simulink model "PruebaSS"  (R2022a)
settings: Solver=VariableStepAuto  StartTime=0.0  StopTime=inf  RelTol=1e-3
values from neighbouring files (symbols this model uses):
  a = 0.2    [Data.m]
  alturaobst = 0.9    [Data.m]
  b = 0.542    [Data.m]
  Ki = 2.88815347475101    (= 2.88815347475)    [Data.m]
  Kp = 0.135293078315631    (= 0.135293078316)    [Data.m]
  M = [x_new y_new]    [Data.m]
  M_chasis = 3.5    [Data.m]
  M_rueda = 1    [Data.m]
  M_ruedacontacto = 1    [Data.m]
  N = 4365    [GraficasVelocidades.m]    (also in Prueba_Liapunov.m = length(p_X); WaypointsToTrayectory.m = length(X))
  posBordes = [xobstac, yobstac; xp1, yobstac; xp2, yobstac; xobstac, yp1; xobstac, yp2 ... (first row only)    [Data.m]
  pruebaM = WaypointsToTrayectory(prue,div)    [Data.m]
  R = 0.175/2    (= 0.0875)    [Data.m]
  X = M(:,1)    [WaypointsToTrayectory.m]
  x0 = x_ini(1)*factorE    [Data.m]
  x_obj = pos_fin(1)*factorE    [Data.m]
  xobstac = RandomPos(1)    [Data.m]
  Y = M(:, 2)    [WaypointsToTrayectory.m]
  y0 = y_ini(2)*factorE    [Data.m]
  y_obj = pos_fin(2)*factorE    [Data.m]
  yobstac = RandomPos(2)    [Data.m]
  zobstac = RandomPos(3)    [Data.m]
undefined symbols (not defined in the file or in its folder): bloqueobstaculo, Borde11, Borde12, Borde2, Borde3, Borde41, Borde42, Explanada, Kd, plano150g1, plano150g2, plano150g3, plano150g4, Plano150mm, plano150mm2irr, Plano45mm, plano45mm2irr, Plano90mm, Rampa, Rampa21, Rampa22, Rampa31, Rampa32, Rampa33, Rampa4, Rampa51, Rampa52, Rampa53, Terreno, Z
libraries: sm_lib x333, nesl_utility x29, fl_lib x3, slpidlib x2, robotalgslib x2
(part 7 of 7)

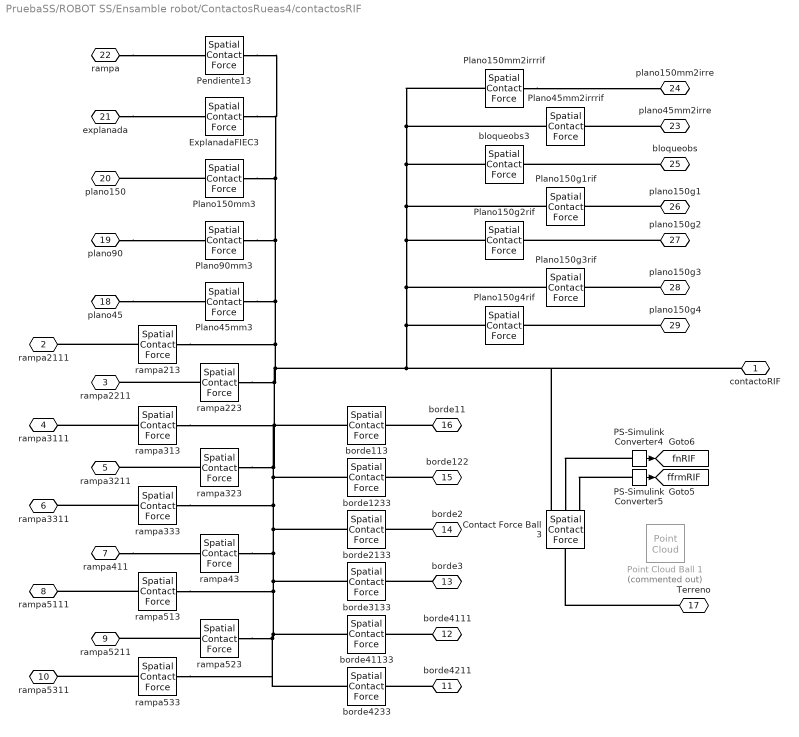
== system PruebaSS/ROBOT SS/Ensamble robot/ContactosRueas4/contactosRIF ==
  Contact Force Ball 3 : sm_lib/Forces and Torques/Spatial Contact Force  SenseContactBaseRotation=off  SenseContactBaseTranslation=off  CoefficientOfDynamicFriction=0.5  CoefficientOfStaticFriction=0.8  NormalDamping=1000  NormalDampingUnits=N/(m/s)  SenseContactSignal=off  NormalStiffness=1000000  NormalStiffnessUnits=N/m  FrictionalCriticalVelocity=1e-3  FrictionalCriticalVelocityUnits=m/s  ZeroCrossDetectContactStartAndEnd=off  SenseContactFollowerRotation=off  SenseContactFollowerTranslation=off  FrictionType=SmoothStickSlip  SenseFrictionalForceMagnitude=on  SenseNormalForceMagnitude=on  NormalForceType=SmoothSpringDamper  SenseNormalVelocity=off  SenseSeparationDistance=off  SenseTangentialVelocity=off  NormalTransitionRegionWidth=1e-4  NormalTransitionRegionWidthUnits=m
  ExplanadaFIEC3 : sm_lib/Forces and Torques/Spatial Contact Force  SenseContactBaseRotation=off  SenseContactBaseTranslation=off  CoefficientOfDynamicFriction=0.3  CoefficientOfStaticFriction=0.5  NormalDamping=1e3  NormalDampingUnits=N/(m/s)  SenseContactSignal=off  NormalStiffness=1e6  NormalStiffnessUnits=N/m  FrictionalCriticalVelocity=1e-3  FrictionalCriticalVelocityUnits=m/s  ZeroCrossDetectContactStartAndEnd=off  SenseContactFollowerRotation=off  SenseContactFollowerTranslation=off  FrictionType=SmoothStickSlip  SenseFrictionalForceMagnitude=off  SenseNormalForceMagnitude=off  NormalForceType=SmoothSpringDamper  SenseNormalVelocity=off  SenseSeparationDistance=off  SenseTangentialVelocity=off  NormalTransitionRegionWidth=1e-4  NormalTransitionRegionWidthUnits=m
  PS-Simulink Converter4 : nesl_utility/PS-Simulink Converter  PhysicalDomain=network_engine_domain  SubClassName=ps_output  LeftPortType=input  RightPortType=output  PseudoPeriodic=off  Frequencies=[]  VectorFormat=inherit  Unit=inherit  AffineConversion=off
      settings: SourceProductBaseCode=SS,PW,VE
  PS-Simulink Converter5 : nesl_utility/PS-Simulink Converter  PhysicalDomain=network_engine_domain  SubClassName=ps_output  LeftPortType=input  RightPortType=output  PseudoPeriodic=off  Frequencies=[]  VectorFormat=inherit  Unit=inherit  AffineConversion=off
      settings: SourceProductBaseCode=SS,PW,VE
  Pendiente13 : sm_lib/Forces and Torques/Spatial Contact Force  SenseContactBaseRotation=off  SenseContactBaseTranslation=off  CoefficientOfDynamicFriction=0.3  CoefficientOfStaticFriction=0.5  NormalDamping=1e3  NormalDampingUnits=N/(m/s)  SenseContactSignal=off  NormalStiffness=1e6  NormalStiffnessUnits=N/m  FrictionalCriticalVelocity=1e-3  FrictionalCriticalVelocityUnits=m/s  ZeroCrossDetectContactStartAndEnd=off  SenseContactFollowerRotation=off  SenseContactFollowerTranslation=off  FrictionType=SmoothStickSlip  SenseFrictionalForceMagnitude=off  SenseNormalForceMagnitude=off  NormalForceType=SmoothSpringDamper  SenseNormalVelocity=off  SenseSeparationDistance=off  SenseTangentialVelocity=off  NormalTransitionRegionWidth=1e-4  NormalTransitionRegionWidthUnits=m
  Plano150g1rif : sm_lib/Forces and Torques/Spatial Contact Force  SenseContactBaseRotation=off  SenseContactBaseTranslation=off  CoefficientOfDynamicFriction=0.3  CoefficientOfStaticFriction=0.5  NormalDamping=1e3  NormalDampingUnits=N/(m/s)  SenseContactSignal=off  NormalStiffness=1e6  NormalStiffnessUnits=N/m  FrictionalCriticalVelocity=1e-3  FrictionalCriticalVelocityUnits=m/s  ZeroCrossDetectContactStartAndEnd=off  SenseContactFollowerRotation=off  SenseContactFollowerTranslation=off  FrictionType=SmoothStickSlip  SenseFrictionalForceMagnitude=off  SenseNormalForceMagnitude=off  NormalForceType=SmoothSpringDamper  SenseNormalVelocity=off  SenseSeparationDistance=off  SenseTangentialVelocity=off  NormalTransitionRegionWidth=1e-4  NormalTransitionRegionWidthUnits=m
  Plano150g2rif : sm_lib/Forces and Torques/Spatial Contact Force  SenseContactBaseRotation=off  SenseContactBaseTranslation=off  CoefficientOfDynamicFriction=0.3  CoefficientOfStaticFriction=0.5  NormalDamping=1e3  NormalDampingUnits=N/(m/s)  SenseContactSignal=off  NormalStiffness=1e6  NormalStiffnessUnits=N/m  FrictionalCriticalVelocity=1e-3  FrictionalCriticalVelocityUnits=m/s  ZeroCrossDetectContactStartAndEnd=off  SenseContactFollowerRotation=off  SenseContactFollowerTranslation=off  FrictionType=SmoothStickSlip  SenseFrictionalForceMagnitude=off  SenseNormalForceMagnitude=off  NormalForceType=SmoothSpringDamper  SenseNormalVelocity=off  SenseSeparationDistance=off  SenseTangentialVelocity=off  NormalTransitionRegionWidth=1e-4  NormalTransitionRegionWidthUnits=m
  Plano150g3rif : sm_lib/Forces and Torques/Spatial Contact Force  SenseContactBaseRotation=off  SenseContactBaseTranslation=off  CoefficientOfDynamicFriction=0.3  CoefficientOfStaticFriction=0.5  NormalDamping=1e3  NormalDampingUnits=N/(m/s)  SenseContactSignal=off  NormalStiffness=1e6  NormalStiffnessUnits=N/m  FrictionalCriticalVelocity=1e-3  FrictionalCriticalVelocityUnits=m/s  ZeroCrossDetectContactStartAndEnd=off  SenseContactFollowerRotation=off  SenseContactFollowerTranslation=off  FrictionType=SmoothStickSlip  SenseFrictionalForceMagnitude=off  SenseNormalForceMagnitude=off  NormalForceType=SmoothSpringDamper  SenseNormalVelocity=off  SenseSeparationDistance=off  SenseTangentialVelocity=off  NormalTransitionRegionWidth=1e-4  NormalTransitionRegionWidthUnits=m
  Plano150g4rif : sm_lib/Forces and Torques/Spatial Contact Force  SenseContactBaseRotation=off  SenseContactBaseTranslation=off  CoefficientOfDynamicFriction=0.3  CoefficientOfStaticFriction=0.5  NormalDamping=1e3  NormalDampingUnits=N/(m/s)  SenseContactSignal=off  NormalStiffness=1e6  NormalStiffnessUnits=N/m  FrictionalCriticalVelocity=1e-3  FrictionalCriticalVelocityUnits=m/s  ZeroCrossDetectContactStartAndEnd=off  SenseContactFollowerRotation=off  SenseContactFollowerTranslation=off  FrictionType=SmoothStickSlip  SenseFrictionalForceMagnitude=off  SenseNormalForceMagnitude=off  NormalForceType=SmoothSpringDamper  SenseNormalVelocity=off  SenseSeparationDistance=off  SenseTangentialVelocity=off  NormalTransitionRegionWidth=1e-4  NormalTransitionRegionWidthUnits=m
  Plano150mm2irrrif : sm_lib/Forces and Torques/Spatial Contact Force  SenseContactBaseRotation=off  SenseContactBaseTranslation=off  CoefficientOfDynamicFriction=0.3  CoefficientOfStaticFriction=0.5  NormalDamping=1e3  NormalDampingUnits=N/(m/s)  SenseContactSignal=off  NormalStiffness=1e6  NormalStiffnessUnits=N/m  FrictionalCriticalVelocity=1e-3  FrictionalCriticalVelocityUnits=m/s  ZeroCrossDetectContactStartAndEnd=off  SenseContactFollowerRotation=off  SenseContactFollowerTranslation=off  FrictionType=SmoothStickSlip  SenseFrictionalForceMagnitude=off  SenseNormalForceMagnitude=off  NormalForceType=SmoothSpringDamper  SenseNormalVelocity=off  SenseSeparationDistance=off  SenseTangentialVelocity=off  NormalTransitionRegionWidth=1e-4  NormalTransitionRegionWidthUnits=m
  Plano150mm3 : sm_lib/Forces and Torques/Spatial Contact Force  SenseContactBaseRotation=off  SenseContactBaseTranslation=off  CoefficientOfDynamicFriction=0.3  CoefficientOfStaticFriction=0.5  NormalDamping=1e3  NormalDampingUnits=N/(m/s)  SenseContactSignal=off  NormalStiffness=1e6  NormalStiffnessUnits=N/m  FrictionalCriticalVelocity=1e-3  FrictionalCriticalVelocityUnits=m/s  ZeroCrossDetectContactStartAndEnd=off  SenseContactFollowerRotation=off  SenseContactFollowerTranslation=off  FrictionType=SmoothStickSlip  SenseFrictionalForceMagnitude=off  SenseNormalForceMagnitude=off  NormalForceType=SmoothSpringDamper  SenseNormalVelocity=off  SenseSeparationDistance=off  SenseTangentialVelocity=off  NormalTransitionRegionWidth=1e-4  NormalTransitionRegionWidthUnits=m
  Plano45mm2irrrif : sm_lib/Forces and Torques/Spatial Contact Force  SenseContactBaseRotation=off  SenseContactBaseTranslation=off  CoefficientOfDynamicFriction=0.3  CoefficientOfStaticFriction=0.5  NormalDamping=1e3  NormalDampingUnits=N/(m/s)  SenseContactSignal=off  NormalStiffness=1e6  NormalStiffnessUnits=N/m  FrictionalCriticalVelocity=1e-3  FrictionalCriticalVelocityUnits=m/s  ZeroCrossDetectContactStartAndEnd=off  SenseContactFollowerRotation=off  SenseContactFollowerTranslation=off  FrictionType=SmoothStickSlip  SenseFrictionalForceMagnitude=off  SenseNormalForceMagnitude=off  NormalForceType=SmoothSpringDamper  SenseNormalVelocity=off  SenseSeparationDistance=off  SenseTangentialVelocity=off  NormalTransitionRegionWidth=1e-4  NormalTransitionRegionWidthUnits=m
  Plano45mm3 : sm_lib/Forces and Torques/Spatial Contact Force  SenseContactBaseRotation=off  SenseContactBaseTranslation=off  CoefficientOfDynamicFriction=0.3  CoefficientOfStaticFriction=0.5  NormalDamping=1e3  NormalDampingUnits=N/(m/s)  SenseContactSignal=off  NormalStiffness=1e6  NormalStiffnessUnits=N/m  FrictionalCriticalVelocity=1e-3  FrictionalCriticalVelocityUnits=m/s  ZeroCrossDetectContactStartAndEnd=off  SenseContactFollowerRotation=off  SenseContactFollowerTranslation=off  FrictionType=SmoothStickSlip  SenseFrictionalForceMagnitude=off  SenseNormalForceMagnitude=off  NormalForceType=SmoothSpringDamper  SenseNormalVelocity=off  SenseSeparationDistance=off  SenseTangentialVelocity=off  NormalTransitionRegionWidth=1e-4  NormalTransitionRegionWidthUnits=m
  Plano90mm3 : sm_lib/Forces and Torques/Spatial Contact Force  SenseContactBaseRotation=off  SenseContactBaseTranslation=off  CoefficientOfDynamicFriction=0.3  CoefficientOfStaticFriction=0.5  NormalDamping=1e3  NormalDampingUnits=N/(m/s)  SenseContactSignal=off  NormalStiffness=1e6  NormalStiffnessUnits=N/m  FrictionalCriticalVelocity=1e-3  FrictionalCriticalVelocityUnits=m/s  ZeroCrossDetectContactStartAndEnd=off  SenseContactFollowerRotation=off  SenseContactFollowerTranslation=off  FrictionType=SmoothStickSlip  SenseFrictionalForceMagnitude=off  SenseNormalForceMagnitude=off  NormalForceType=SmoothSpringDamper  SenseNormalVelocity=off  SenseSeparationDistance=off  SenseTangentialVelocity=off  NormalTransitionRegionWidth=1e-4  NormalTransitionRegionWidthUnits=m
  Point Cloud Ball 1 : sm_lib/Curves and Surfaces/Point Cloud  Commented=on  CoordinatesMatrix=rueda_ptcld  CoordinatesMatrixUnits=m  GraphicType=MarkerCloud  GraphicSphereRadius=0.001  GraphicSphereRadiusUnits=m  GraphicVisPropType=SimpleVisualProperties  GraphicDiffuseColor=[1 0 0]  GraphicOpacity=1  GraphicSpecularColor=[0.5 0.5 0.5 1.0]  GraphicAmbientColor=[0.15 0.15 0.15 1.0]  GraphicEmissiveColor=[0.0 0.0 0.0 1.0]  GraphicShininess=75
      settings: SourceProductBaseCode=MS
  bloqueobs3 : sm_lib/Forces and Torques/Spatial Contact Force  SenseContactBaseRotation=off  SenseContactBaseTranslation=off  CoefficientOfDynamicFriction=0.3  CoefficientOfStaticFriction=0.5  NormalDamping=1e3  NormalDampingUnits=N/(m/s)  SenseContactSignal=off  NormalStiffness=1e6  NormalStiffnessUnits=N/m  FrictionalCriticalVelocity=1e-3  FrictionalCriticalVelocityUnits=m/s  ZeroCrossDetectContactStartAndEnd=off  SenseContactFollowerRotation=off  SenseContactFollowerTranslation=off  FrictionType=SmoothStickSlip  SenseFrictionalForceMagnitude=off  SenseNormalForceMagnitude=off  NormalForceType=SmoothSpringDamper  SenseNormalVelocity=off  SenseSeparationDistance=off  SenseTangentialVelocity=off  NormalTransitionRegionWidth=1e-4  NormalTransitionRegionWidthUnits=m
  borde{113,1233,2133,3133,4233,41133} (6 alike) : sm_lib/Forces and Torques/Spatial Contact Force  SenseContactBaseRotation=off  SenseContactBaseTranslation=off  CoefficientOfDynamicFriction=0.3  CoefficientOfStaticFriction=0.5  NormalDamping=1e3  NormalDampingUnits=N/(m/s)  SenseContactSignal=off  NormalStiffness=1e6  NormalStiffnessUnits=N/m  FrictionalCriticalVelocity=1e-3  FrictionalCriticalVelocityUnits=m/s  ZeroCrossDetectContactStartAndEnd=off  SenseContactFollowerRotation=off  SenseContactFollowerTranslation=off  FrictionType=SmoothStickSlip  SenseFrictionalForceMagnitude=off  SenseNormalForceMagnitude=off  NormalForceType=SmoothSpringDamper  SenseNormalVelocity=off  SenseSeparationDistance=off  SenseTangentialVelocity=off  NormalTransitionRegionWidth=1e-4  NormalTransitionRegionWidthUnits=m
  rampa{43,213,223,313,323,333,513,523,533} (9 alike) : sm_lib/Forces and Torques/Spatial Contact Force  SenseContactBaseRotation=off  SenseContactBaseTranslation=off  CoefficientOfDynamicFriction=0.3  CoefficientOfStaticFriction=0.5  NormalDamping=1e3  NormalDampingUnits=N/(m/s)  SenseContactSignal=off  NormalStiffness=1e6  NormalStiffnessUnits=N/m  FrictionalCriticalVelocity=1e-3  FrictionalCriticalVelocityUnits=m/s  ZeroCrossDetectContactStartAndEnd=off  SenseContactFollowerRotation=off  SenseContactFollowerTranslation=off  FrictionType=SmoothStickSlip  SenseFrictionalForceMagnitude=off  SenseNormalForceMagnitude=off  NormalForceType=SmoothSpringDamper  SenseNormalVelocity=off  SenseSeparationDistance=off  SenseTangentialVelocity=off  NormalTransitionRegionWidth=1e-4  NormalTransitionRegionWidthUnits=m
  contactoRIF : PMIOPort  Side=Left
  rampa2111 : PMIOPort  Port=2  Side=Left
  rampa2211 : PMIOPort  Port=3  Side=Left
  rampa3111 : PMIOPort  Port=4  Side=Left
  rampa3211 : PMIOPort  Port=5  Side=Left
  rampa3311 : PMIOPort  Port=6  Side=Left
  rampa411 : PMIOPort  Port=7  Side=Left
  rampa5111 : PMIOPort  Port=8  Side=Left
  rampa5211 : PMIOPort  Port=9  Side=Left
  rampa5311 : PMIOPort  Port=10  Side=Left
  borde4211 : PMIOPort  Port=11  Side=Right
  borde4111 : PMIOPort  Port=12  Side=Right
  borde3 : PMIOPort  Port=13  Side=Right
  borde2 : PMIOPort  Port=14  Side=Right
  borde122 : PMIOPort  Port=15  Side=Right
  borde11 : PMIOPort  Port=16  Side=Right
  Terreno : PMIOPort  Port=17  Side=Right
  plano45 : PMIOPort  Port=18  Side=Right
  plano90 : PMIOPort  Port=19  Side=Right
  plano150 : PMIOPort  Port=20  Side=Right
  explanada : PMIOPort  Port=21  Side=Right
  rampa : PMIOPort  Port=22  Side=Right
  plano45mm2irre : PMIOPort  Port=23  Side=Right
  plano150mm2irre : PMIOPort  Port=24  Side=Right
  bloqueobs : PMIOPort  Port=25  Side=Right
  plano150g1 : PMIOPort  Port=26  Side=Right
  plano150g2 : PMIOPort  Port=27  Side=Right
  plano150g3 : PMIOPort  Port=28  Side=Right
  plano150g4 : PMIOPort  Port=29  Side=Right
  tag scope: ffrmRIF=global, fnRIF=global
  wires:
  PS-Simulink Converter5/1 -> [ffrmRIF]
  PS-Simulink Converter4/1 -> [fnRIF]
  connections:
  Plano150mm2irrrif/RConn1 -- bloqueobs3/RConn1 -- Plano150g1rif/RConn1 -- Plano150g2rif/RConn1 -- Plano150g3rif/RConn1 -- Plano150g4rif/RConn1 -- rampa213/RConn1 -- Plano90mm3/RConn1 -- Pendiente13/RConn1 -- ExplanadaFIEC3/RConn1 -- Plano150mm3/RConn1 -- Plano45mm3/RConn1 -- rampa333/RConn1 -- borde2133/LConn1 -- borde3133/LConn1 -- borde41133/LConn1 -- borde4233/LConn1 -- rampa533/RConn1 -- rampa523/RConn1 -- rampa513/RConn1 -- rampa43/RConn1 -- borde1233/LConn1 -- rampa323/RConn1 -- borde113/LConn1 -- rampa313/RConn1 -- rampa223/RConn1 -- Contact Force Ball 3/RConn1 -- contactoRIF/RConn1 -- Plano45mm2irrrif/RConn1
  Plano150mm3/LConn1 -- plano150/RConn1
  plano90/RConn1 -- Plano90mm3/LConn1
  plano45/RConn1 -- Plano45mm3/LConn1
  rampa/RConn1 -- Pendiente13/LConn1
  PS-Simulink Converter4/LConn1 -- Contact Force Ball 3/RConn2
  explanada/RConn1 -- ExplanadaFIEC3/LConn1
  Terreno/RConn1 -- Contact Force Ball 3/LConn1
  PS-Simulink Converter5/LConn1 -- Contact Force Ball 3/RConn3
  rampa213/LConn1 -- rampa2111/RConn1
  rampa333/LConn1 -- rampa3311/RConn1
  rampa513/LConn1 -- rampa5111/RConn1
  rampa533/LConn1 -- rampa5311/RConn1
  rampa523/LConn1 -- rampa5211/RConn1
  rampa223/LConn1 -- rampa2211/RConn1
  rampa313/LConn1 -- rampa3111/RConn1
  rampa411/RConn1 -- rampa43/LConn1
  rampa323/LConn1 -- rampa3211/RConn1
  borde4211/RConn1 -- borde4233/RConn1
  borde122/RConn1 -- borde1233/RConn1
  borde3/RConn1 -- borde3133/RConn1
  borde11/RConn1 -- borde113/RConn1
  borde4111/RConn1 -- borde41133/RConn1
  borde2/RConn1 -- borde2133/RConn1
  plano150g4/RConn1 -- Plano150g4rif/LConn1
  bloqueobs/RConn1 -- bloqueobs3/LConn1
  plano150g2/RConn1 -- Plano150g2rif/LConn1
  plano150g1/RConn1 -- Plano150g1rif/LConn1
  plano150g3/RConn1 -- Plano150g3rif/LConn1
  Plano150mm2irrrif/LConn1 -- plano150mm2irre/RConn1
  plano45mm2irre/RConn1 -- Plano45mm2irrrif/LConn1

== system PruebaSS/ROBOT SS/Ensamble robot/Tapa/Frontal ==
  Cylindrical Solid : sm_lib/Body Elements/Cylindrical Solid  GraphicAmbientColor=[0.15 0.15 0.15 1.0]  BasedOnType=Density  CenterOfMass=[0 0 0]  CenterOfMassUnits=m  GraphicDiffuseColor=[0.5 0.5 0.5]  CylinderLength=0.3  CylinderLengthUnits=m  CylinderRadius=0.1  CylinderRadiusUnits=m  Density=1000  DensityUnits=kg/m^3  DoExposeReferenceFrame=on  GraphicEmissiveColor=[0.0 0.0 0.0 1.0]  ExportEntireGeometry=off  SerializedFrames=<Frames><Frame><Id>Frame1</Id><Value><Name>F1</Name><Origin><Source>GeometricFeature</Source><FeatureName>top curve</FeatureName></Origin><PrimaryAxis><DefinedDirection>+X</DefinedDirection><Source>GeometricFeature</Source><SourceDirection>+Z</SourceDirection><FeatureName>top curve</FeatureName></PrimaryAxis><SecondaryAxis><DefinedDirection>-Z</DefinedDirection><Source>ReferenceFrame</Source><SourceDirection>+X</SourceDirection><FeatureName></FeatureName></SecondaryAxis></Value></Frame></Frames>  MarkerShape=Sphere  MarkerSize=10  GraphicType=None  InertiaType=CalculateFromGeometry  Mass=1  MassUnits=kg  MomentsOfInertia=[1 1 1]  MomentsOfInertiaUnits=kg*m^2  GraphicOpacity=1.0  ProductsOfInertia=[0 0 0]  ProductsOfInertiaUnits=kg*m^2  GraphicShininess=75  GraphicSpecularColor=[0.5 0.5 0.5 1.0]  GraphicVisPropType=SimpleVisualProperties
  Cylindrical Solid1 : sm_lib/Body Elements/Cylindrical Solid  GraphicAmbientColor=[0.15 0.15 0.15 1.0]  BasedOnType=Density  CenterOfMass=[0 0 0]  CenterOfMassUnits=m  GraphicDiffuseColor=[0.5 0.5 0.5]  CylinderLength=0.1  CylinderLengthUnits=m  CylinderRadius=0.1  CylinderRadiusUnits=m  Density=1000  DensityUnits=kg/m^3  DoExposeReferenceFrame=on  GraphicEmissiveColor=[0.0 0.0 0.0 1.0]  ExportEntireGeometry=off  SerializedFrames=<Frames/>  MarkerShape=Sphere  MarkerSize=10  GraphicType=None  InertiaType=CalculateFromGeometry  Mass=1  MassUnits=kg  MomentsOfInertia=[1 1 1]  MomentsOfInertiaUnits=kg*m^2  GraphicOpacity=1.0  ProductsOfInertia=[0 0 0]  ProductsOfInertiaUnits=kg*m^2  GraphicShininess=75  GraphicSpecularColor=[0.5 0.5 0.5 1.0]  GraphicVisPropType=SimpleVisualProperties
  Conn1 : PMIOPort  Side=Right
  connections:
  Cylindrical Solid1/RConn1 -- Cylindrical Solid/LConn1
  Cylindrical Solid/RConn1 -- Conn1/RConn1

== system PruebaSS/Sistema de Control/Planificación Local/Cinemática Inversa/Direct-Kinematics ==
  wl : Inport
  wr : Inport  Port=2
  w : Inport  Port=3
  Constant : Constant  Value=[540 241 2*pi/3]
  Constant1 : Constant  Value=0.08
  Constant2 : Constant  Value=2*a
  Constant3 : Constant  Value=b
  Integrator2 : Integrator
  Integrator3 : Integrator  InitialCondition=x0
  Integrator4 : Integrator  InitialCondition=y0
  MATLAB Function : MATLAB Function  TreatAsAtomicUnit=on
  Mux : Mux  Inputs=3
  Pose : Outport
  wires:
  Mux/1 -> Pose/1
  Integrator4/1 -> Mux/2
  Constant3/1 -> MATLAB Function/5(a)
  MATLAB Function/3(o) -> Mux/3
  MATLAB Function/1(xp) -> Integrator3/1
  Integrator3/1 -> Mux/1
  Integrator2/1 -> MATLAB Function/6(or)
  w/1 -> Integrator2/1
  wr/1 -> MATLAB Function/1(wr)
  Constant1/1 -> MATLAB Function/3(r)
  MATLAB Function/2(yp) -> Integrator4/1
  Constant2/1 -> MATLAB Function/4(c)
  wl/1 -> MATLAB Function/2(wl)

== system PruebaSS/Sistema de Control/Planificación Local/Cinemática Inversa/Inverse-Kinematics1 ==
  v : Inport
  w : Inport  Port=2
  Gain : Gain  Gain=b/2
  Gain1 : Gain  Gain=1/R
  Gain2 : Gain  Gain=1/R
  Sum : Sum  Inputs=|+-
  Sum1 : Sum  Inputs=|++
  wL : Outport
  wR : Outport  Port=2
  wires:
  Gain/1 -> Sum1/2, Sum/2
  Sum/1 -> Gain1/1
  Gain1/1 -> wL/1
  Gain2/1 -> wR/1
  v/1 -> Sum1/1, Sum/1
  Sum1/1 -> Gain2/1
  w/1 -> Gain/1

== system PruebaSS/Sistema de Control/Planificación Local/Cinemática Inversa/Inverse-Kinematics2 ==
  v : Inport
  w : Inport  Port=2
  Constant : Constant  Value=R
  Constant1 : Constant  Value=b
  MATLAB Function : MATLAB Function  TreatAsAtomicUnit=on
  wL : Outport
  wR : Outport  Port=2
  wires:
  Constant1/1 -> MATLAB Function/2(R)
  Constant/1 -> MATLAB Function/3(b)
  MATLAB Function/2(wR) -> wR/1
  MATLAB Function/1(wL) -> wL/1
  w/1 -> MATLAB Function/4(w)
  v/1 -> MATLAB Function/1(v)

== system PruebaSS/Sistema de Control/Planificación Local/Motion Planning/IdentificarRampa ==
  R_Pose : Inport
  Display : Display
  MATLAB Function1 : MATLAB Function  TreatAsAtomicUnit=on
  Rampa1 : Constant  Value=[192.8, 260]
  Rampa2 : Constant  Value=[200.3, 273]
  Rampa3 : Constant  Value=[204.6, 289]
  d : Outport
  i : Outport  Port=2
  wires:
  R_Pose/1 -> Display/1, MATLAB Function1/1(R_Pose)
  Rampa1/1 -> MATLAB Function1/2(Rampa_P)
  MATLAB Function1/1(d) -> d/1
  Rampa2/1 -> MATLAB Function1/3(Rampa2)
  MATLAB Function1/2(i) -> i/1
  Rampa3/1 -> MATLAB Function1/4(Rampa3)

== system PruebaSS/Sistema de Control/Planificación Local/Motion Planning/Seguidor de Camino ==
  Robot_Pose : Inport
  Global_Waypoints : Inport  Port=2
  Clock : Clock
  Constant : Constant  Value=0.5
  Display : Display
  Display1 : Display
  Display2 : Display
  Goal : Constant  Value=[x_obj ,y_obj]
  Perfil de aceleración y desaceleración : MATLAB Function  TreatAsAtomicUnit=on
  Pure  Pursuit : robotalgslib/Pure Pursuit  DesiredLinearVelocity=1.38  MaxAngularVelocity=pi  LookaheadDistance=.08  TargetDirPort=off  SimulateUsing=Code generation
  Reductor de Velocidad en Curvas : Subsystem
  Saturation : Saturate  UpperLimit=2.5  LowerLimit=-2.5
  Subsystem1 : Subsystem
  To Workspace : ToWorkspace  VariableName=RobotPose  SampleTime=-1
  hold : Subsystem
  t1 : Constant  Value=0.5
  atgoal : Outport
  W : Outport  Port=2
  v : Outport  Port=3
  wires:
  Subsystem1/2(atgoal) -> Display/1, atgoal/1
  hold/1(deaccelStartTime) -> Perfil de aceleración y desaceleración/5(deaccelStartTime)
  Robot_Pose/1 -> Pure  Pursuit/1, To Workspace/1, Subsystem1/3(Pose)
  Subsystem1/1(deAcc) -> hold/1(deAcc)
  Pure  Pursuit/1 -> Subsystem1/1(linearV), Perfil de aceleración y desaceleración/1(linVel)
  Clock/1 -> Perfil de aceleración y desaceleración/2(t)
  Constant/1 -> Perfil de aceleración y desaceleración/4(accel)
  t1/1 -> Perfil de aceleración y desaceleración/3(t1)
  Global_Waypoints/1 -> Pure  Pursuit/2
  Goal/1 -> Subsystem1/2(Goal)
  Perfil de aceleración y desaceleración/1(lin_Vel_out) -> Display1/1, Reductor de Velocidad en Curvas/1(v_in)
  Pure  Pursuit/2 -> Display2/1, Perfil de aceleración y desaceleración/6(w)
  Perfil de aceleración y desaceleración/2(w_out) -> Reductor de Velocidad en Curvas/2(w_in)
  Reductor de Velocidad en Curvas/2(w_out) -> Saturation/1
  Reductor de Velocidad en Curvas/1(v_out) -> v/1
  Saturation/1 -> W/1

== system PruebaSS/Sistema de Control/Planificación Local/Motion Planning/Seguidor de Camino/Reductor de Velocidad en Curvas ==
  v_in : Inport
  w_in : Inport  Port=2
  Constant1 : Constant  Value=2.5
  Demux : Demux  Outputs=2
  Gain : Gain  Gain=0.01
  GreaterThan : RelationalOperator  Operator=<=  OutDataTypeStr=boolean  RndMeth=Simplest  InputSameDT=off
  Mux : Mux  Inputs=2
  Mux1 : Mux  Inputs=2
  Switch1 : Switch  Threshold=1  SaturateOnIntegerOverflow=off  InputSameDT=off
  v_out : Outport
  w_out : Outport  Port=2
  wires:
  Demux/1 -> v_out/1
  w_in/1 -> Mux1/2, Mux/2, GreaterThan/1
  Mux/1 -> Switch1/1
  GreaterThan/1 -> Switch1/2
  Demux/2 -> w_out/1
  Mux1/1 -> Switch1/3
  v_in/1 -> Gain/1, Mux/1
  Switch1/1 -> Demux/1
  Constant1/1 -> GreaterThan/2
  Gain/1 -> Mux1/1

== system PruebaSS/Sistema de Control/Planificación Local/Motion Planning/Seguidor de Camino/Subsystem1 ==
  linearV : Inport
  Goal : Inport  Port=2
  Pose : Inport  Port=3
  Add : Sum
  Constant : Constant  Value=2* 1
  Constant1 : Constant  Value=2
  Gain : Gain
  GreaterThan : RelationalOperator  OutDataTypeStr=boolean  RndMeth=Simplest  InputSameDT=off
  GreaterThan1 : RelationalOperator  Operator=>  OutDataTypeStr=boolean  RndMeth=Simplest  InputSameDT=off
  NOT : Logic  Operator=NOT  IconShape=distinctive  AllPortsSameDT=off  OutDataTypeStr=boolean
  Product : Product  Inputs=*/
  Square : Math  Operator=square
  Unit Delay : UnitDelay  SampleTime=-1  HasFrameUpgradeWarning=on
  check-goal : Subsystem
  deAcc : Outport
  atgoal : Outport  Port=2
  wires:
  Gain/1 -> Add/2
  linearV/1 -> Square/1
  Unit Delay/1 -> atgoal/1
  Pose/1 -> check-goal/1(Pose)
  NOT/1 -> Unit Delay/1
  GreaterThan/1 -> deAcc/1
  Square/1 -> Product/1
  GreaterThan1/1 -> NOT/1
  Product/1 -> Add/1
  Add/1 -> GreaterThan/2
  Constant1/1 -> Gain/1, GreaterThan1/2
  Constant/1 -> Product/2
  check-goal/1(distanceGoal) -> GreaterThan1/1, GreaterThan/1
  Goal/1 -> check-goal/2(Goal)

== system PruebaSS/Sistema de Control/Planificación Local/Motion Planning/Seguidor de Camino/hold ==
  deAcc : Inport
  Constant9 : Constant  Value=inf
  NOT1 : Logic  Operator=NOT  IconShape=distinctive  AllPortsSameDT=off  OutDataTypeStr=boolean
  StopTime : Subsystem
  Switch3 : Switch  Criteria=u2 > Threshold  SaturateOnIntegerOverflow=off  InputSameDT=off
  Unit Delay1 : UnitDelay  SampleTime=-1  HasFrameUpgradeWarning=on
  deaccelStartTime : Outport
  wires:
  deAcc/1 -> NOT1/1
  Constant9/1 -> Switch3/3
  NOT1/1 -> Unit Delay1/1, StopTime/1(Enable)
  Switch3/1 -> deaccelStartTime/1
  StopTime/1(DeAccelTime) -> Switch3/1
  Unit Delay1/1 -> Switch3/2

== system PruebaSS/Sistema de Control/Planificación Local/Motion Planning/Seguidor de Camino/Subsystem1/check-goal ==
  Pose : Inport
  Goal : Inport  Port=2
  MATLAB Function : MATLAB Function  TreatAsAtomicUnit=on
  Scope : Scope
  Selector : Selector  InputPortWidth=3  IndexOptions=Index vector (dialog)  Indices=[1 2]  OutputSizes=1
  distanceGoal : Outport
  wires:
  MATLAB Function/1(distanceGoal) -> Scope/1, distanceGoal/1
  Goal/1 -> MATLAB Function/2(goal)
  Selector/1 -> MATLAB Function/1(posexy)
  Pose/1 -> Selector/1

== system PruebaSS/Sistema de Control/Planificación Local/Motion Planning/Seguidor de Camino/hold/StopTime ==
  Enable : Inport
  Clock : Clock
  Constant2 : Constant
  Display : Display
  Enabled Subsystem1 : Subsystem  TreatAsAtomicUnit=on
      settings: MinAlgLoopOccurrences=on
  Switch : Switch  Criteria=u2 > Threshold  SaturateOnIntegerOverflow=off  InputSameDT=off
  Unit Delay : UnitDelay  SampleTime=-1  HasFrameUpgradeWarning=on
  DeAccelTime : Outport
  wires:
  Constant2/1 -> Enabled Subsystem1/1(In1)
  Clock/1 -> Switch/3
  Unit Delay/1 -> Switch/1, DeAccelTime/1, Display/1
  Switch/1 -> Unit Delay/1
  Enable/1 -> Enabled Subsystem1/Enable
  Enabled Subsystem1/1(Out1) -> Switch/2

== system PruebaSS/Sistema de Control/Planificación Local/Motion Planning/Seguidor de Camino/hold/StopTime/Enabled Subsystem1 ==
  In1 : Inport
  Enable : EnablePort
  Out1 : Outport
  wires:
  In1/1 -> Out1/1

== matlab function PruebaSS/Sistema de Control/Planificación Local/Motion Planning/Seguidor de Camino/Perfil de aceleración y desaceleración ==
  data: linVel input; t input; t1 input; lin_Vel_out output; accel input; deaccelStartTime input; w input; w_out output
function [lin_Vel_out, w_out]= fcn(linVel,t,t1,accel,deaccelStartTime, w)
% Function to create a trapezoidal profile for desired linear
% velocity

t2 = linVel/accel + t1;
t3 = deaccelStartTime + 0.2;
tf = linVel/accel + t3;

if t>=t1 && t<t2 
    lin_Vel_out = accel*(t-t1);
     w_out = w;

elseif t>=t2 && t < t3 
    lin_Vel_out = linVel;
    w_out= w;

elseif t>= t3 && t < tf 
    lin_Vel_out = linVel-accel*(t-t3);
    w_out= w-accel*(t-t3);

else
    lin_Vel_out = 0;  w_out = w;  
end


end

== matlab function PruebaSS/Sistema de Control/Planificación Local/Cinemática Inversa/Inverse-Kinematics2/MATLAB Function ==
  data: v input; R input; b input; wL output; w input; wR output
function [wL,wR] = fcn(v, R, b, w)

wL= (v - (b/2)*w )/R;


wR= (v + (b/2)*w )/R;

== matlab function PruebaSS/Sensores/Percepción/Subsystem1/Sensor Ultrasónico 3 ==
  data: R_Pose input; r input; d_in input; phi input; Pose_Obs input; val output
function val = fcn(R_Pose, r, d_in, phi, Pose_Obs)
%% valor por defecto


%% CALCULO POSICIÓN DEL SENSOR CON RESPECTO AL ROBOT

x_Sensor= R_Pose(1) + d_in*cos(R_Pose(3)+phi);
y_Sensor= R_Pose(2) + d_in*sin(R_Pose(3)+phi);

%% CÁLCULO DE DISTANCIA y ÁNGULO ENTRE EL SENSOR Y LOS PUNTOS DEL OBSTÁCULO
N=length(Pose_Obs);
d= [0; 0; 0; 0; 0; 0; 0; 0; 0];
angulo= [0; 0; 0; 0; 0; 0; 0; 0; 0];
for i= 1:N
    d_SyO= sqrt((x_Sensor-Pose_Obs(i,1))^2 + (y_Sensor - Pose_Obs(i,2))^2);
    betha = atan2((Pose_Obs(i,2) - y_Sensor),(Pose_Obs(i,1)- x_Sensor));
    phi1= betha - R_Pose(3);
    d(i)= d_SyO;
    angulo(i)= phi1;

end

valores = [0; 0; 0; 0; 0; 0; 0; 0; 0];
for j= 1:N

    dj= d(j);
    phijj=angulo(j);
    if (abs(phijj - phi) <= r)
        valores(j) = dj;
    else
        valores(j) = 1000;

    end

end


val = min(valores);

end




%% CALCULO DEL ANGULO DEL VECTOR QUE FORMA LA POS DEL SENSOR Y EL OBSTÁCULO

== matlab function PruebaSS/Sensores/Percepción/Subsystem1/Sensor Ultrasónico 4 ==
  data: R_Pose input; r input; d_in input; phi input; Pose_Obs input; val output
function val = fcn(R_Pose, r, d_in, phi, Pose_Obs)
%% valor por defecto


%% CALCULO POSICIÓN DEL SENSOR CON RESPECTO AL ROBOT

x_Sensor= R_Pose(1) + d_in*cos(R_Pose(3)+phi);
y_Sensor= R_Pose(2) + d_in*sin(R_Pose(3)+phi);

%% CÁLCULO DE DISTANCIA y ÁNGULO ENTRE EL SENSOR Y LOS PUNTOS DEL OBSTÁCULO
N=length(Pose_Obs);
d= [0; 0; 0; 0; 0; 0; 0; 0; 0];
angulo= [0; 0; 0; 0; 0; 0; 0; 0; 0];
for i= 1:N
    d_SyO= sqrt((x_Sensor-Pose_Obs(i,1))^2 + (y_Sensor - Pose_Obs(i,2))^2);
    betha = atan2((Pose_Obs(i,2) - y_Sensor),(Pose_Obs(i,1)- x_Sensor));
    phi1= betha - R_Pose(3);
    d(i)= d_SyO;
    angulo(i)= phi1;

end

valores = [0; 0; 0; 0; 0; 0; 0; 0; 0];
for j= 1:N

    dj= d(j);
    phijj=angulo(j);
    if (abs(phijj - phi) <= r)
        valores(j) = dj;
    else
        valores(j) = 1000;

    end

end


val = min(valores);

end




%% CALCULO DEL ANGULO DEL VECTOR QUE FORMA LA POS DEL SENSOR Y EL OBSTÁCULO

== matlab function PruebaSS/Sensores/Percepción/Subsystem1/Sensor Ultrasónico 5 ==
  data: R_Pose input; r input; d_in input; phi input; Pose_Obs input; val output
function val = fcn(R_Pose, r, d_in, phi, Pose_Obs)
%% valor por defecto


%% CALCULO POSICIÓN DEL SENSOR CON RESPECTO AL ROBOT

x_Sensor= R_Pose(1) + d_in*cos(R_Pose(3)+phi);
y_Sensor= R_Pose(2) + d_in*sin(R_Pose(3)+phi);

%% CÁLCULO DE DISTANCIA y ÁNGULO ENTRE EL SENSOR Y LOS PUNTOS DEL OBSTÁCULO
N=length(Pose_Obs);
d= [0; 0; 0; 0; 0; 0; 0; 0; 0];
angulo= [0; 0; 0; 0; 0; 0; 0; 0; 0];
for i= 1:N
    d_SyO= sqrt((x_Sensor-Pose_Obs(i,1))^2 + (y_Sensor - Pose_Obs(i,2))^2);
    betha = atan2((Pose_Obs(i,2) - y_Sensor),(Pose_Obs(i,1)- x_Sensor));
    phi1= betha - R_Pose(3);
    d(i)= d_SyO;
    angulo(i)= phi1;

end

valores = [0; 0; 0; 0; 0; 0; 0; 0; 0];
for j= 1:N

    dj= d(j);
    phijj=angulo(j);
    if (abs(phijj - phi) <= r)
        valores(j) = dj;
    else
        valores(j) = 1000;

    end

end


val = min(valores);

end




%% CALCULO DEL ANGULO DEL VECTOR QUE FORMA LA POS DEL SENSOR Y EL OBSTÁCULO

== matlab function PruebaSS/Sensores/Percepción/Subsystem1/Sensor Ultrasónico 6 ==
  data: R_Pose input; r input; d_in input; phi input; Pose_Obs input; val output
function val = fcn(R_Pose, r, d_in, phi, Pose_Obs)
%% valor por defecto


%% CALCULO POSICIÓN DEL SENSOR CON RESPECTO AL ROBOT

x_Sensor= R_Pose(1) + d_in*cos(R_Pose(3)+phi);
y_Sensor= R_Pose(2) + d_in*sin(R_Pose(3)+phi);

%% CÁLCULO DE DISTANCIA y ÁNGULO ENTRE EL SENSOR Y LOS PUNTOS DEL OBSTÁCULO
N=length(Pose_Obs);
d= [0; 0; 0; 0; 0; 0; 0; 0; 0];
angulo= [0; 0; 0; 0; 0; 0; 0; 0; 0];
for i= 1:N
    d_SyO= sqrt((x_Sensor-Pose_Obs(i,1))^2 + (y_Sensor - Pose_Obs(i,2))^2);
    betha = atan2((Pose_Obs(i,2) - y_Sensor),(Pose_Obs(i,1)- x_Sensor));
    phi1= betha - R_Pose(3);
    d(i)= d_SyO;
    angulo(i)= phi1;

end

valores = [0; 0; 0; 0; 0; 0; 0; 0; 0];
for j= 1:N

    dj= d(j);
    phijj=angulo(j);
    if (abs(phijj - phi) <= r)
        valores(j) = dj;
    else
        valores(j) = 1000;

    end

end


val = min(valores);

end




%% CALCULO DEL ANGULO DEL VECTOR QUE FORMA LA POS DEL SENSOR Y EL OBSTÁCULO

== matlab function PruebaSS/Sensores/Percepción/Subsystem1/Sensor Ultrasónico 7 ==
  data: R_Pose input; r input; d_in input; phi input; Pose_Obs input; val output
function val = fcn(R_Pose, r, d_in, phi, Pose_Obs)
%% valor por defecto


%% CALCULO POSICIÓN DEL SENSOR CON RESPECTO AL ROBOT

x_Sensor= R_Pose(1) + d_in*cos(R_Pose(3)+phi);
y_Sensor= R_Pose(2) + d_in*sin(R_Pose(3)+phi);

%% CÁLCULO DE DISTANCIA y ÁNGULO ENTRE EL SENSOR Y LOS PUNTOS DEL OBSTÁCULO
N=length(Pose_Obs);
d= [0; 0; 0; 0; 0; 0; 0; 0; 0];
angulo= [0; 0; 0; 0; 0; 0; 0; 0; 0];
for i= 1:N
    d_SyO= sqrt((x_Sensor-Pose_Obs(i,1))^2 + (y_Sensor - Pose_Obs(i,2))^2);
    betha = atan2((Pose_Obs(i,2) - y_Sensor),(Pose_Obs(i,1)- x_Sensor));
    phi1= betha - R_Pose(3);
    d(i)= d_SyO;
    angulo(i)= phi1;

end

valores = [0; 0; 0; 0; 0; 0; 0; 0; 0];
for j= 1:N

    dj= d(j);
    phijj=angulo(j);
    if (abs(phijj - phi) <= r)
        valores(j) = dj;
    else
        valores(j) = 1000;

    end

end


val = min(valores);

end




%% CALCULO DEL ANGULO DEL VECTOR QUE FORMA LA POS DEL SENSOR Y EL OBSTÁCULO

== matlab function PruebaSS/Sistema de Control/Planificación Local/Evasión_Obstaculos/Identificar Obstáculo ==
  data: On_Off output; dis input
function On_Off = fcn(dis)

if (dis(4) <= 1.5 || dis(3) <= 1.5|| dis(5) <=1.5 || dis(1) <= 1.5|| dis(2) <= 1.5|| dis(6) <=1.5 || dis(7) <=1.5)

    On_Off =0;
else
    On_Off=1;
end

== matlab function PruebaSS/ROBOT SS/DOF/theta ==
  data: Q input; oz output
function oz  = fcn(Q)
out = quat2eul(Q');
oz = out(1);

end

== matlab function PruebaSS/Sensores/Percepción/Subsystem1/Sensor Ultrasónico 9 ==
  data: R_Pose input; d_out output; d_in input; phi input; Pose_Obs input
function d_out = fcn(R_Pose, d_in, phi, Pose_Obs)
%% valor por defecto


%% CALCULO POSICIÓN DEL SENSOR CON RESPECTO AL ROBOT

x_Sensor= R_Pose(1) + d_in*cos(R_Pose(3)+phi);
y_Sensor= R_Pose(2) + d_in*sin(R_Pose(3)+phi);

%% CALCULO DE DISTANCIA ENTRE EL SENSOR Y EL OBSTÁCULO

d_SyO= sqrt((x_Sensor-Pose_Obs(1))^2 + (y_Sensor - Pose_Obs(2))^2);

%% CALCULO DEL ANGULO DEL VECTOR QUE FORMA LA POS DEL SENSOR Y EL OBSTÁCULO

betha = atan((Pose_Obs(2) - R_Pose(2))/(Pose_Obs(1)- R_Pose(1)));

phi1= betha - R_Pose(3);

if (abs(phi1 - phi) <= 0.5)

    if(d_SyO<= 8)
        d_out = d_SyO;
    else
        d_out = 1000;
    end

   
else
    d_out = 1000;
end

== matlab function PruebaSS/Sistema de Control/Planificación Local/Motion Planning/IdentificarRampa/MATLAB Function1 ==
  data: R_Pose input; d output; Rampa_P input; Rampa2 input; i output; Rampa3 input
function [d, i]= fcn(R_Pose, Rampa_P, Rampa2, Rampa3)


y1= sqrt((R_Pose(1)-Rampa_P(1))^2 + (R_Pose(2)-Rampa_P(2))^2);
y2= sqrt((R_Pose(1)-Rampa2(1))^2 + (R_Pose(2)-Rampa2(2))^2);
y3= sqrt((R_Pose(1)-Rampa3(1))^2 + (R_Pose(2)-Rampa3(2))^2);

if y1<= 10 || y2<=10 || y3<=10

    d= 0;

else
    d=1;

end

if y1<y2 && y1<y3

    i=1;
elseif y2<y1 && y2<y3

    i=2;
elseif y3<y2 && y3<y1
    i=3;
else
    i=0;

end

== matlab function PruebaSS/ROBOT SS/Promedio ==
  data: wr output; wl output; w1 input; w2 input; w3 input; w4 input
function [wr, wl] = Promedio(w1,w2,w3,w4)

wr= (w1+w2)/(2);
wl= (w3+w4)/(2);

== matlab function PruebaSS/ROBOT SS/Subsystem/Rot 2 eul ==
  data: z output; R input
function z  = fcn(R)
out = rotm2eul(R);
z = out(1);
end

== matlab function PruebaSS/ROBOT SS/Subsystem/Vlineal ==
  data: vx input; v output; vy input
function v = fcn(vx, vy)

v = sqrt((vx)^2 + (vy)^2);
end

== matlab function PruebaSS/Sistema de Control/Planificación Local/Evasión_Obstaculos/Esquema de Evasión ==
  data: dis input; wr_out output; wl_out output
function [wr_out,wl_out] = fcn(dis)
w=10;

if (dis(4)< 1.5)

    if(dis(3) < 2 && dis(5)> 1)
        %giro fuerte a la derecha
        wr_out= -w;
        wl_out= w ;

    elseif dis(5)<2 && dis(3)> 1
        %giro fuerte a la izquierda
        wr_out= w;
        wl_out= -w;

    else
        %Por defecto gira por la izq

        %giro fuerte a la izquierda
        wr_out= w;
        wl_out= -w;
    end

elseif dis(5)< 0.2
    %giro medio a la izquierda
        wr_out= w;
        wl_out= w/2;
elseif dis(6)< 0.2

    wr_out= w;
    wl_out= w*0.75;



elseif dis(7)< 0.2
    %giro suave a la izquierda
        wr_out= w;
        wl_out= w*0.8;

else
    wr_out= w;
    wl_out= w;    
end

== matlab function PruebaSS/Sensores/Percepción/Subsystem1/Sensor Ultrasónico 2 ==
  data: R_Pose input; r input; d_in input; phi input; Pose_Obs input; val output
function val = fcn(R_Pose, r, d_in, phi, Pose_Obs)
%% valor por defecto


%% CALCULO POSICIÓN DEL SENSOR CON RESPECTO AL ROBOT

x_Sensor= R_Pose(1) + d_in*cos(R_Pose(3)+phi);
y_Sensor= R_Pose(2) + d_in*sin(R_Pose(3)+phi);

%% CÁLCULO DE DISTANCIA y ÁNGULO ENTRE EL SENSOR Y LOS PUNTOS DEL OBSTÁCULO
N=length(Pose_Obs);
d= [0; 0; 0; 0; 0; 0; 0; 0; 0];
angulo= [0; 0; 0; 0; 0; 0; 0; 0; 0];
for i= 1:N
    d_SyO= sqrt((x_Sensor-Pose_Obs(i,1))^2 + (y_Sensor - Pose_Obs(i,2))^2);
    betha = atan2((Pose_Obs(i,2) - y_Sensor),(Pose_Obs(i,1)- x_Sensor));
    phi1= betha - R_Pose(3);
    d(i)= d_SyO;
    angulo(i)= phi1;

end

valores = [0; 0; 0; 0; 0; 0; 0; 0; 0];
for j= 1:N

    dj= d(j);
    phijj=angulo(j);
    if (abs(phijj - phi) <= r)
        valores(j) = dj;
    else
        valores(j) = 1000;

    end

end


val = min(valores);

end




%% CALCULO DEL ANGULO DEL VECTOR QUE FORMA LA POS DEL SENSOR Y EL OBSTÁCULO

== matlab function PruebaSS/Sensores/Percepción/Subsystem1/Sensor Ultrasónico 1 ==
  data: R_Pose input; r input; d_in input; phi input; Pose_Obs input; val output
function val = fcn(R_Pose, r, d_in, phi, Pose_Obs)
%% valor por defecto


%% CALCULO POSICIÓN DEL SENSOR CON RESPECTO AL ROBOT

x_Sensor= R_Pose(1) + d_in*cos(R_Pose(3)+phi);
y_Sensor= R_Pose(2) + d_in*sin(R_Pose(3)+phi);

%% CÁLCULO DE DISTANCIA y ÁNGULO ENTRE EL SENSOR Y LOS PUNTOS DEL OBSTÁCULO
N=length(Pose_Obs);
d= [0; 0; 0; 0; 0; 0; 0; 0; 0];
angulo= [0; 0; 0; 0; 0; 0; 0; 0; 0];
for i= 1:N
    d_SyO= sqrt((x_Sensor-Pose_Obs(i,1))^2 + (y_Sensor - Pose_Obs(i,2))^2);
    betha = atan2((Pose_Obs(i,2) - y_Sensor),(Pose_Obs(i,1)- x_Sensor));
    phi1= betha - R_Pose(3);
    d(i)= d_SyO;
    angulo(i)= phi1;

end

valores = [0; 0; 0; 0; 0; 0; 0; 0; 0];
for j= 1:N

    dj= d(j);
    phijj=angulo(j);
    if (abs(phijj - phi) <= r)
        valores(j) = dj;
    else
        valores(j) = 1000;

    end

end


val = min(valores);

end




%% CALCULO DEL ANGULO DEL VECTOR QUE FORMA LA POS DEL SENSOR Y EL OBSTÁCULO

== matlab function PruebaSS/Sistema de Control/Planificación Local/Cinemática Inversa/Direct-Kinematics/MATLAB Function ==
  data: xp output; yp output; wr input; wl input; r input; c input; a input; o output; or input
function [xp,yp,o] = fcn(wr,wl,r,c,a, or)

o= or;

v1= c*cos(o) - 2*a*sin(o);
v2= c*cos(o) + 2*a*sin(o);
v3= c*sin(o) + 2*a*cos(o);
v4= c*sin(o) - 2*a*cos(o);

xp=(r/(2*c))*(v1*wr+v2*wl);
yp= (r/(2*c))*(v3*wr+v4*wl);

== matlab function PruebaSS/Sistema de Control/Planificación Local/Motion Planning/Seguidor de Camino/Subsystem1/check-goal/MATLAB Function ==
  data: posexy input; distanceGoal output; goal input
function distanceGoal  = fcn( posexy, goal)

distanceGoal = sqrt(((goal(1)-posexy(1))^2)+ ((goal(2)-posexy(2))^2) );
end
